simulink model "bol1_ejer5_grafica1"  (R2021a)
settings: Solver=VariableStepAuto  StartTime=0.0  StopTime=10.0  RelTol=1e-3
settings Model: Creator=andrea  LastModifiedBy=andrea

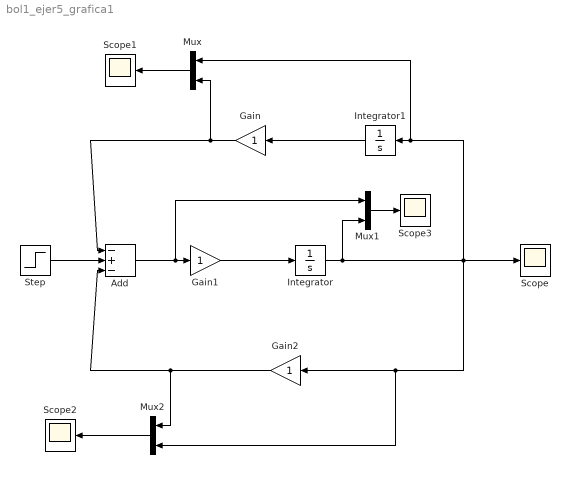
== system bol1_ejer5_grafica1 ==
  Add : Sum  Inputs=-+-
  Gain : Gain
  Gain1 : Gain
  Gain2 : Gain
  Integrator : Integrator
  Integrator1 : Integrator
  Mux : Mux  Inputs=2
  Mux1 : Mux  Inputs=2
  Mux2 : Mux  Inputs=2
  Scope{,1..3} (4 alike) : Scope
  Step : Step  SampleTime=0
  wires:
  Step/1 -> Add/2
  Gain/1 -> Mux/2, Add/1
  Integrator1/1 -> Gain/1
  Gain2/1 -> Mux2/1, Add/3
  Add/1 -> Mux1/1, Gain1/1
  Gain1/1 -> Integrator/1
  Integrator/1 -> Gain2/1, Mux2/2, Scope/1, Mux/1, Integrator1/1, Mux1/2
  Mux/1 -> Scope1/1
  Mux2/1 -> Scope2/1
  Mux1/1 -> Scope3/1
